simulink library "message_holder_lib"  (R2021a)
settings: Solver=VariableStepAuto  StartTime=0.0  StopTime=10.0  RelTol=1e-3
undefined symbols (not defined in the file or in its folder): DiscIntNeverNeededParam
settings Model: Creator=Rahul Subramanian  LastModifiedBy=Rahul Subramanian

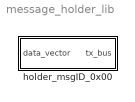
== system message_holder_lib ==
  holder_msgID_0x00 : Subsystem  mask{u_p=0}

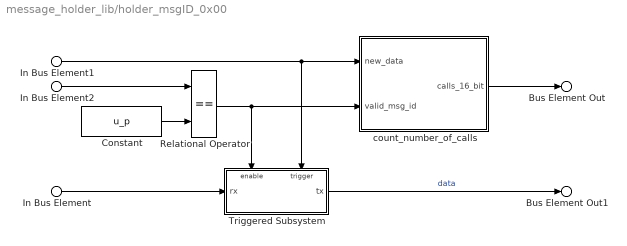
== system message_holder_lib/holder_msgID_0x00 ==
  In Bus Element : Inport  PortName=data_vector  Element=data_vector
  In Bus Element1 : Inport  PortName=data_vector  Element=new_data
  In Bus Element2 : Inport  PortName=data_vector  Element=msg_id
  Constant : Constant  Value=u_p
  Relational Operator : RelationalOperator  Operator===  OutDataTypeStr=boolean  RndMeth=Simplest
  Triggered Subsystem : Subsystem  TreatAsAtomicUnit=on
  count_number_of_calls : Subsystem
  Bus Element Out : Outport  PortName=tx_bus  Element=calls_16_bit
  Bus Element Out1 : Outport  PortName=tx_bus  Element=data
  wires:
  In Bus Element1/1 -> Triggered Subsystem/Trigger, count_number_of_calls/1(new_data)
  In Bus Element/1 -> Triggered Subsystem/1(rx)
  Relational Operator/1 -> Triggered Subsystem/Enable, count_number_of_calls/2(valid_msg_id)
  In Bus Element2/1 -> Relational Operator/1
  Constant/1 -> Relational Operator/2
  Triggered Subsystem/1(tx) -> Bus Element Out1/1  "data"
  count_number_of_calls/1(calls_16_bit) -> Bus Element Out/1

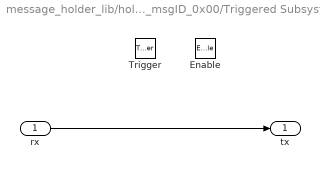
== system message_holder_lib/holder_msgID_0x00/Triggered Subsystem ==
  rx : Inport
  Enable : EnablePort
  Trigger : TriggerPort  VariantControl=(inherit)
  tx : Outport
  wires:
  rx/1 -> tx/1

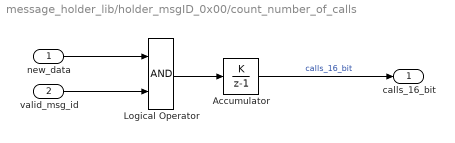
== system message_holder_lib/holder_msgID_0x00/count_number_of_calls ==
  new_data : Inport
  valid_msg_id : Inport  Port=2
  Accumulator : DiscreteIntegrator  IntegratorMethod=Accumulation: Forward Euler  SampleTime=-1  OutDataTypeStr=uint16  ICPrevOutput=DiscIntNeverNeededParam  ICPrevScaledInput=DiscIntNeverNeededParam
  Logical Operator : Logic  AllPortsSameDT=off  OutDataTypeStr=boolean
  calls_16_bit : Outport
  wires:
  Logical Operator/1 -> Accumulator/1
  valid_msg_id/1 -> Logical Operator/2
  new_data/1 -> Logical Operator/1
  Accumulator/1 -> calls_16_bit/1  "calls_16_bit"
